simulink model "Temporal8"  (R2020a)
settings: Solver=VariableStepAuto  StartTime=0.0  StopTime=1.0  RelTol=1e-3
settings Model: Creator=86188  LastModifiedBy=bzhan
settings DataIOCC: ReturnWorkspaceOutputs=off
settings DebuggingCC: ArithmeticOperatorsInVariantConditions=warning
settings SFSimCC: SimUseLocalCustomCode=off  CustomCodeUndefinedFunction=UseInterfaceOnly
settings RTWCC: RTWUseLocalCustomCode=off

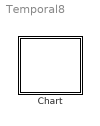
== system Temporal8 ==
  Chart : Stateflow chart  TreatAsAtomicUnit=on

== stateflow chart Temporal8/Chart ==
  settings: updateMethod=DISCRETE  sampleTime=0.1
  state A
    en:f("en_A");
    x=1;
    A -> A [order 1] : {f("du_A");
        | x=x+1;}
  state B
    en:f("en_B")
    du:f("du_B");
  (default) -> A
  A -> B [order 1] : after(3,tick)[x>=5]
  B -> A : after(3,tick)
  data: s function_input; x local
  function f(s):
    | function f(s)
    |   fprintf(s+"\n");
